simulink model "custom_springs_3"  (R2026a)
settings: Solver=VariableStepAuto  StopTime=15  MaxStep=1e-1  AbsTol=1e-3  EnableMultiTasking=on
InitFcn:
  | warning off Simulink:SL_MatchingFromNotFound
  | m=1;
  | b=1;
  | k=1;
libraries: fl_lib x16, nesl_utility x4
Description:
  | Copyright 2014-2026 The MathWorks, Inc.
settings Model: Creator=tegel  LastModifiedBy=smiller
settings DataIOCC: SignalLoggingSaveFormat=ModelDataLogs
settings OptimizationCC: InitFltsAndDblsToZero=on
settings DebuggingCC: SaveWithParameterizedLinksMsg=none  UnderspecifiedInitializationDetection=Classic
settings HardwareCC: ProdHWDeviceType=32-bit Generic
settings GRTTargetCC: TargetFcnLib=ansi_tfl_tmw.mat  CombineOutputUpdateFcns=off  GRTInterface=on
settings SimscapeCC: SimscapeNormalizeSystem=off  SimscapeNominalValues="[{\"value\":\"1\",\"unit\":\"A\"},{\"value\":\"1\",\"unit\":\"bar\"},{\"value\":\"1\",\"unit\":\"cm^2\"},{\"value\":\"1\",\"unit\":\"cm^3/s\"},{\"value\":\"1\",\"unit\":\"kJ/kg\"},{\"value\":\"1\",\"unit\":\"kW\"},{\"value\":\"1\",\"unit\":\"l\"},{\"value\":\"1\",\"unit\":\"N\"},{\"value\":\"1\",\"unit\":\"N*m\"},{\"value\":\"1\",\"unit\":\"V\"}]"  SimscapeLogType=none  SimscapeLogDataHistory=5000.0

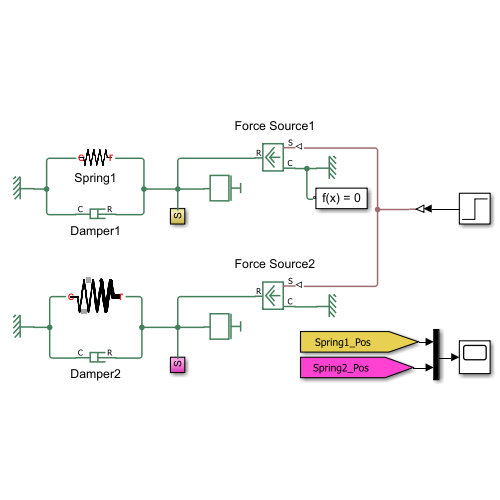
[thumbnail: Simulink's stored preview of the top-level diagram]
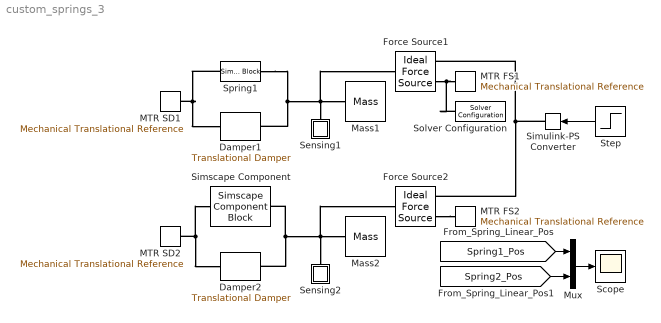
== system custom_springs_3 ==
  Damper1 : fl_lib/Mechanical/Translational Elements/Translational Damper  D=b N/(m/s)  v_specify=off  v_priority=High  v=0 m/s  v_nominal_specify=off  v_nominal_value=1  v_nominal_unit=m/s  f_specify=off  f_priority=High  f=0 N  f_nominal_specify=off  f_nominal_value=1  f_nominal_unit=N
  Damper2 : fl_lib/Mechanical/Translational Elements/Translational Damper  D=b N/(m/s)  v_specify=off  v_priority=High  v=0 m/s  v_nominal_specify=off  v_nominal_value=1  v_nominal_unit=m/s  f_specify=off  f_priority=High  f=0 N  f_nominal_specify=off  f_nominal_value=1  f_nominal_unit=N
  Force Source1 : fl_lib/Mechanical/Mechanical Sources/Ideal Force Source
  Force Source2 : fl_lib/Mechanical/Mechanical Sources/Ideal Force Source
  MTR FS1 : fl_lib/Mechanical/Translational Elements/Mechanical Translational Reference
  MTR FS2 : fl_lib/Mechanical/Translational Elements/Mechanical Translational Reference
  MTR SD1 : fl_lib/Mechanical/Translational Elements/Mechanical Translational Reference
  MTR SD2 : fl_lib/Mechanical/Translational Elements/Mechanical Translational Reference
  Mass1 : fl_lib/Mechanical/Translational Elements/Mass  mass=m kg  num_ports=foundation.enum.numPorts2.one  v_specify=on  v_priority=High  v=0 m/s  v_nominal_specify=off  v_nominal_value=1  v_nominal_unit=m/s  f_specify=off  f_priority=High  f=0 N  f_nominal_specify=off  f_nominal_value=1  f_nominal_unit=N
  Mass2 : fl_lib/Mechanical/Translational Elements/Mass  mass=m kg  num_ports=foundation.enum.numPorts2.one  v_specify=on  v_priority=High  v=0 m/s  v_nominal_specify=off  v_nominal_value=1  v_nominal_unit=m/s  f_specify=off  f_priority=High  f=0 N  f_nominal_specify=off  f_nominal_value=1  f_nominal_unit=N
  Mux : Mux  Inputs=2
  Scope : Scope
      settings: TimeSpan=15  ActiveDisplayYMinimum=0  ActiveDisplayYMaximum=2.5
  Sensing1 : Subsystem
  Sensing2 : Subsystem
  Simscape Component : SimscapeComponentBlock  SourceFile=CustomSprings.SpringRegions  ComponentPath=CustomSprings.SpringRegions  ComponentVariants=CustomSprings.SpringRegions  ComponentVariantNames=SpringRegions  ClassName=SpringRegions  SchemaVersion=1  k=1 N/m  k1=1 N/m^3  xc=0.2 m  v_specify=off  v_priority=None  v=0 m/s  v_nominal_specify=off  v_nominal_value=1  v_nominal_unit=m/s  f_specify=off  f_priority=None  f=0 N  f_nominal_specify=off  f_nominal_value=1  f_nominal_unit=N  x_specify=off  x_priority=None  x=0 m  x_nominal_specify=off  x_nominal_value=1  x_nominal_unit=m
      settings: CopyFcn=simscape.sscblock.internal.componentBlockCallback(gcbh,'COPY')  PreCopyFcn=simscape.sscblock.internal.componentBlockCallback(gcbh,'PRECOPY')  PreDeleteFcn=simscape.sscblock.internal.componentBlockCallback(gcbh,'PREDELETE')
      mask Type: Spring (Regions)
  Simulink-PS Converter : nesl_utility/Simulink-PS Converter  PhysicalDomain=network_engine_domain  SubClassName=ps_input  LeftPortType=input  RightPortType=output  PseudoPeriodic=off  Frequencies=[]  NoiseDistribution=none  NoiseParameters=[]  Unit=1  AffineConversion=off  FilteringAndDerivatives=provide  SimscapeFilterOrder=1  InputFilterTimeConstant=.001  UdotUserProvided=0
  Solver Configuration : nesl_utility/Solver Configuration  PhysicalDomain=network_engine_domain  SubClassName=solver  LeftPortType=input  RightPortType=generic  Tones=[]  Harmonics=[]  SimulateNoise=off  Profile=off  UseLocalSampling=off  EnableSwitchedLinearOptims=on  FrequencyDomain=off  UseCCode=off  RelTol=0.001  AbsTol=1e-06  MinStep=1e-09  ToWorkspace=off  RevertToSquareIcSolve=off  NumHomotopyIterations=100  PhasorMode=off  PhasorModeNumHarmonics=1  ConsistencySolver=NEWTON_FTOL  CanonicalOrdering=UNORDERED  OptimizeIntermediates=UNOPTIMIZED  IndexReductionMethod=DerivativeReplacement  DoDC=off  ResidualTolerance=1e-9  ConsistencyTolSource=GLOBAL  ConsistencyAbsTol=0.001  ConsistencyRelTol=0.001  ConsistencyTolFactor=0.001  UseLocalSolver=off  LocalSolverChoice=NE_BACKWARD_EULER_ADVANCER  ResolveIndetEquations=on  FunctionEvalNumThread=1  LocalSolverSampleTime=.001  DoFixedCost=off  MaxNonlinIter=3  MaxModeIter=2  ComputeImpulses=off  ImpulseIterations=2  LinearAlgebra=Sparse  LinearAlgebraNumThread=0  EquationFormulation=NE_TIME_EF  DelaysMemoryBudget=1024  AutomaticFiltering=on  FilteringTimeConstant=0.001  PartitionStorageMethod=AS_NEEDED  PartitionMemoryBudget=1024  PartitionMethod=FAST  MultibodyUseLocalSolver=off  MultibodyLocalSolverChoice=ODE1  MultibodyLocalSolverSampleTime=0.001
  Spring1 : SimscapeComponentBlock  SourceFile=CustomSprings.SpringLinear  ComponentPath=CustomSprings.SpringLinear  ComponentVariants=CustomSprings.SpringLinear  ComponentVariantNames=SpringLinear  ClassName=SpringLinear  SchemaVersion=1  k=1 N/m  v_specify=off  v_priority=None  v=0 m/s  v_nominal_specify=off  v_nominal_value=1  v_nominal_unit=m/s  f_specify=off  f_priority=None  f=0 N  f_nominal_specify=off  f_nominal_value=1  f_nominal_unit=N  x_specify=off  x_priority=None  x=0 m  x_nominal_specify=off  x_nominal_value=1  x_nominal_unit=m
      settings: CopyFcn=simscape.sscblock.internal.componentBlockCallback(gcbh,'COPY')  PreCopyFcn=simscape.sscblock.internal.componentBlockCallback(gcbh,'PRECOPY')  PreDeleteFcn=simscape.sscblock.internal.componentBlockCallback(gcbh,'PREDELETE')
      mask Type: Spring
  Step : Step  FinalValue=2  SampleTime=0
  wires:
  Mux/1 -> Scope/1
  [Spring1_Pos] -> Mux/1
  [Spring2_Pos] -> Mux/2
  Step/1 -> Simulink-PS Converter/1
  connections:
  Simulink-PS Converter/RConn1 -- Force Source2/RConn1 -- Force Source1/RConn1
  Force Source1/RConn2 -- Solver Configuration/RConn1 -- MTR FS1/LConn1
  MTR SD1/LConn1 -- Spring1/LConn1 -- Damper1/RConn1
  Damper1/LConn1 -- Spring1/RConn1 -- Sensing1/LConn1 -- Mass1/LConn1 -- Force Source1/LConn1
  MTR SD2/LConn1 -- Simscape Component/LConn1 -- Damper2/RConn1
  Damper2/LConn1 -- Simscape Component/RConn1 -- Sensing2/LConn1 -- Force Source2/LConn1 -- Mass2/LConn1
  Force Source2/RConn2 -- MTR FS2/LConn1

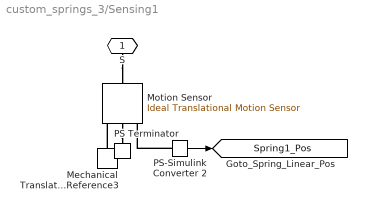
== system custom_springs_3/Sensing1 ==
  Mechanical Translational Reference3 : fl_lib/Mechanical/Translational Elements/Mechanical Translational Reference
  Motion Sensor : fl_lib/Mechanical/Mechanical Sensors/Ideal Translational Motion Sensor  reference=foundation.enum.MeasurementReference.difference  acceleration_port=false  velocity_port=true  position_port=true  offset=0 m
  PS Terminator : fl_lib/Physical Signals/Sinks/PS Terminator
  PS-Simulink Converter 2 : nesl_utility/PS-Simulink Converter  PhysicalDomain=network_engine_domain  SubClassName=ps_output  LeftPortType=input  RightPortType=output  PseudoPeriodic=off  Frequencies=[]  VectorFormat=1-D array  Unit=1  AffineConversion=off
  S : PMIOPort  Side=Left
  tag scope: Spring1_Pos=global
  wires:
  PS-Simulink Converter 2/1 -> [Spring1_Pos]
  connections:
  S/RConn1 -- Motion Sensor/LConn1
  Mechanical Translational Reference3/LConn1 -- Motion Sensor/RConn1
  PS-Simulink Converter 2/LConn1 -- Motion Sensor/RConn3
  Motion Sensor/RConn2 -- PS Terminator/LConn1

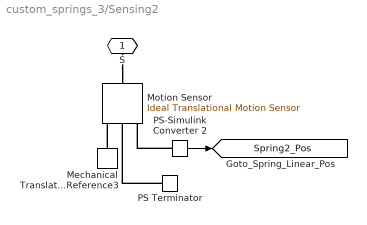
== system custom_springs_3/Sensing2 ==
  Mechanical Translational Reference3 : fl_lib/Mechanical/Translational Elements/Mechanical Translational Reference
  Motion Sensor : fl_lib/Mechanical/Mechanical Sensors/Ideal Translational Motion Sensor  reference=foundation.enum.MeasurementReference.difference  acceleration_port=false  velocity_port=true  position_port=true  offset=0 m
  PS Terminator : fl_lib/Physical Signals/Sinks/PS Terminator
  PS-Simulink Converter 2 : nesl_utility/PS-Simulink Converter  PhysicalDomain=network_engine_domain  SubClassName=ps_output  LeftPortType=input  RightPortType=output  PseudoPeriodic=off  Frequencies=[]  VectorFormat=1-D array  Unit=1  AffineConversion=off
  S : PMIOPort  Side=Left
  tag scope: Spring2_Pos=global
  wires:
  PS-Simulink Converter 2/1 -> [Spring2_Pos]
  connections:
  PS-Simulink Converter 2/LConn1 -- Motion Sensor/RConn3
  PS Terminator/LConn1 -- Motion Sensor/RConn2
  Mechanical Translational Reference3/LConn1 -- Motion Sensor/RConn1
  S/RConn1 -- Motion Sensor/LConn1
